simulink subsystem "Mesurer_la_position_de_la_lame"  (R2020a)
settings: Solver=VariableStepAuto  StartTime=0.0  StopTime=10.0  RelTol=1e-3
values from neighbouring files (symbols this model uses):
  K_pos = 806.5    [default_design_data.mat]    (also in dict.sldd)
  V_consigne = 1.8    [default_design_data.mat]    (also in dict.sldd)
settings Model: Creator=frfoc1  LastModifiedBy=MAGUY18

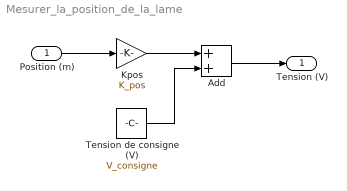
== system Mesurer_la_position_de_la_lame ==
  Position (m) : Inport
  Add : Sum
  Kpos : Gain  Gain=K_pos
  Tension de consigne (V) : Constant  Value=V_consigne
  Tension (V) : Outport
  wires:
  Position (m)/1 -> Kpos/1
  Kpos/1 -> Add/1
  Add/1 -> Tension (V)/1
  Tension de consigne (V)/1 -> Add/2
